simulink model "QAM_cau5"  (R2017b)
settings: Solver=VariableStepAuto  StartTime=0.0  StopTime=10  RelTol=1e-3
settings Model: Creator=admin  LastModifiedBy=admin

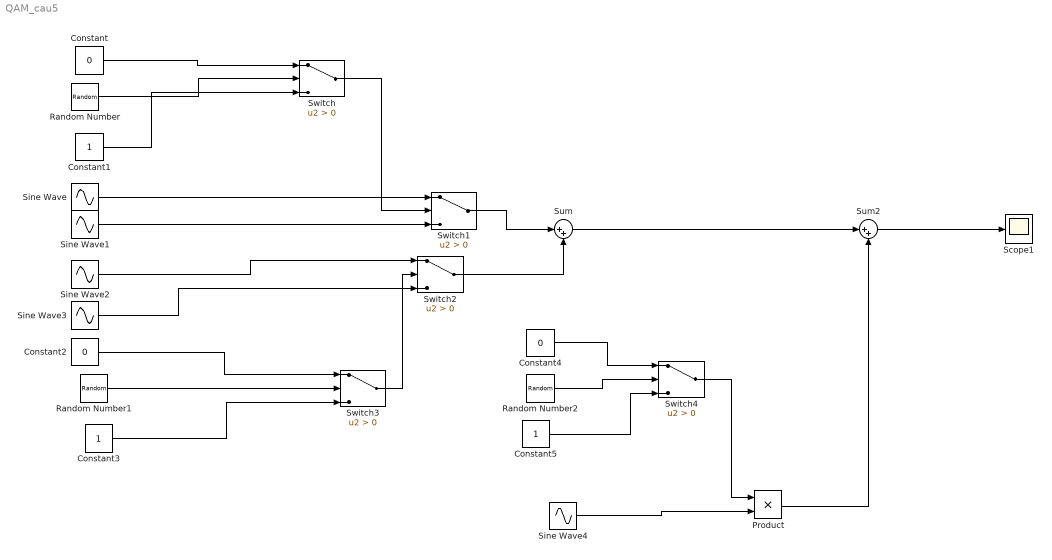
== system QAM_cau5 ==
  Constant : Constant  Value=0
  Constant1 : Constant
  Constant2 : Constant  Value=0
  Constant3 : Constant
  Constant4 : Constant  Value=0
  Constant5 : Constant
  Product : Product
  Random Number : RandomNumber  SampleTime=0.5
  Random Number1 : RandomNumber  SampleTime=0.5
  Random Number2 : RandomNumber  SampleTime=0.5
  Scope1 : Scope
  Sine Wave : Sin  Frequency=4*pi  SampleTime=0.001
  Sine Wave1 : Sin  Frequency=4*pi  Phase=pi  SampleTime=0.0001
  Sine Wave2 : Sin  Frequency=4*pi  Phase=pi/2  SampleTime=0.0001
  Sine Wave3 : Sin  Frequency=4*pi  Phase=3*pi/2  SampleTime=0.0001
  Sine Wave4 : Sin  Frequency=4*pi  SampleTime=0.001
  Sum : Sum  Inputs=|++
  Sum2 : Sum  Inputs=|++
  Switch{,1..4} (5 alike) : Switch  Criteria=u2 > Threshold
  wires:
  Constant/1 -> Switch/1
  Random Number/1 -> Switch/2
  Constant1/1 -> Switch/3
  Switch/1 -> Switch1/2
  Sine Wave/1 -> Switch1/1
  Sine Wave1/1 -> Switch1/3
  Constant2/1 -> Switch3/1
  Random Number1/1 -> Switch3/2
  Constant3/1 -> Switch3/3
  Switch3/1 -> Switch2/2
  Sine Wave2/1 -> Switch2/1
  Sine Wave3/1 -> Switch2/3
  Switch1/1 -> Sum/1
  Switch4/1 -> Product/1
  Random Number2/1 -> Switch4/2
  Constant5/1 -> Switch4/3
  Sine Wave4/1 -> Product/2
  Constant4/1 -> Switch4/1
  Switch2/1 -> Sum/2
  Sum/1 -> Sum2/1
  Product/1 -> Sum2/2
  Sum2/1 -> Scope1/1
